simulink model "Simulacion_trayectoria"  (R2021a)
settings: Solver=VariableStepAuto  StartTime=0.0  StopTime=80  RelTol=1e-3
model workspace: external: MATLAB File G:\My Drive\0. PUCP\Cursos\2020.2\IEE243 - Sistemas de Control\Tarea Academica\Simulacion Robot Movil\cad files\RobotMovil_DataFile.m (data not in the file)
undefined symbols (not defined in the file): smiData, X, xPla, Y, yPla, Z, zPla
libraries: sm_lib x211, nesl_utility x6, simulink x3, fl_lib x3
(part 5 of 5)

== system Simulacion_trayectoria/MODELO CINEMÁTICO ROBOT MOVIL1/RobotMovilBase_2_RIGID/shield_rb_1_RIGID/shield_rb_step_1_RIGID/tc_3528_step_1_RIGID ==
  ReferenceFrame : sm_lib/Frames and Transforms/Reference Frame
  Solid : sm_lib/Body Elements/File Solid  ExtGeomFileName=tc_3528.step_Default_sldprt.STEP  UnitType=FromFile  ExtGeomFileUnits=m  StepReaderType=HEX  ExportConvexHullGeometry=off  InertiaType=Custom  Mass=smiData.Solid(7).mass  MassUnits=kg  CenterOfMass=smiData.Solid(7).CoM  CenterOfMassUnits=mm  MomentsOfInertia=smiData.Solid(7).MoI  MomentsOfInertiaUnits=kg*mm^2  ProductsOfInertia=smiData.Solid(7).PoI  ProductsOfInertiaUnits=kg*mm^2  BasedOnType=DensityFromFile  Density=1000  DensityUnits=kg/m^3  DoExposeReferenceFrame=on  SerializedFrames=<Frames/>  GraphicType=FromGeometry  MarkerShape=Sphere  MarkerSize=10  GraphicVisPropType=SimpleVisualProperties  GraphicDiffuseColor=smiData.Solid(7).color  GraphicSpecularColor=[0.5 0.5 0.5 1.0]  GraphicAmbientColor=[0.15 0.15 0.15 1.0]  GraphicEmissiveColor=[0.0 0.0 0.0 1.0]  GraphicShininess=75  GraphicOpacity=smiData.Solid(7).opacity
  F : PMIOPort  Side=Left
  connections:
  Solid/RConn1 -- ReferenceFrame/RConn1 -- F/RConn1

== matlab function Simulacion_trayectoria/Controlador de Seguimiento de Trayectoria1 ==
  data: xd input; yd input; xdp input; w_ref output; ydp input; x input; y input; u_ref output; phi input
function [w_ref, u_ref] = fcn(xd,yd,xdp,ydp,x,y,phi)

a = 0.147/2;
K1 = 16;%Tes=0.25 seg
K2 = 16;%Tes=0.25 seg
%phi en radianes
xa = x + a*cos(phi);
ya = y + a*sin(phi);
%definimos la matriz M
detM=a;
Minv_11 = a*cos(phi)/detM;
Minv_12 = a*sin(phi)/detM;
Minv_21 = -sin(phi)/detM;
Minv_22 = cos(phi)/detM;
%
av1 = xdp + K1*(xd-xa);
av2 = ydp + K2*(yd-ya);
%
u_ref = Minv_11*av1 + Minv_12*av2;
w_ref = Minv_21*av1 + Minv_22*av2;%está radianes

== matlab function Simulacion_trayectoria/MATLAB Function1 ==
  data: x input; xa output; y input; phi input; ya output
function [xa,ya] = fcn(x,y,phi)

a = 0.147/2;

xa = x + a*cos(phi);
ya = y + a*sin(phi);

== matlab function Simulacion_trayectoria/Trayectoria1 ==
  data: u input; xd output; yd output; xdp output; ydp output
function [xd,yd,xdp,ydp] = fcn(u)
%Son 14 caminos. Si el recorrido total dura 60 segundos, cada camino debe 
%demorar como mucho 4.2857 segundos(aproximamos a 4 segundos). Y dado que
%se desea que en "10 pasos" se pueda cumplir con un trayecto, el tiempo de 
%muestro de este bloque debe ser 0.4segundos.
persistent t
persistent xo
persistent yo
persistent camino_1
persistent camino_2
persistent camino_3
persistent camino_4
persistent camino_5
persistent camino_6
persistent camino_7
persistent camino_8
persistent camino_9
persistent camino_10
persistent camino_11
persistent camino_12
persistent camino_13

if isempty(t)
    t=0;
    xo=0.168;
    yo=0;
    camino_1=true;
    camino_2=true;
    camino_3=true;
    camino_4=true;
    camino_5=true;
    camino_6=true;
    camino_7=true;
    camino_8=true;
    camino_9=true;
    camino_10=true;
    camino_11=true;
    camino_12=true;
    camino_13=true;
end
if camino_1
    xd=xo+0.168*cosd(180-t);
    yd=yo+0.168*sind(180-t);
    %derivada
    xdp=0.168*sind(180-t);
    ydp=0.168*-cosd(180-t);
    if t>=128
        camino_1=false;
        %Añadimos el centro
        xo=xd+0.1*sind(38);
        yo=yd+0.1*cosd(38);
        t=0;
    else
        t = t + 12.8;     
    end
elseif camino_2
    xd=xo+0.1*cosd(-128+t);
    yd=yo+0.1*sind(-128+t);
    %derivada
    xdp=0.1*-sind(-128+t);
    ydp=0.1*cosd(-128+t);
    if t>=78
        camino_2=false;
        %Añadimos el centro
        xo=xd+0.168*sind(40);
        yo=yd-0.168*cosd(40);
        t=0;
    else
        t = t + 7.8;     
    end
elseif camino_3
    xd=xo+0.168*cosd(130-t);
    yd=yo+0.168*sind(130-t);
    %derivada
    xdp=0.168*sind(130-t);
    ydp=0.168*-cosd(130-t);
    if t>=68
        camino_3=false;
        %Añadimos el centro
        xo=xd+0.05*sind(28);
        yo=yd+0.05*cosd(28);
        t=0;
    else
        t = t + 6.8;     
    end   
elseif camino_4
    xd=xo+0.05*cosd(-118+t);
    yd=yo+0.05*sind(-118+t);
    %derivada
    xdp=0.05*-sind(-118+t);
    ydp=0.05*cosd(-118+t);
    if t>=137
        camino_4=false;
        %Añadimos el centro
        xo=xd-0.75*sind(71);
        yo=yd-0.75*cosd(71);
        t=0;
    else
        t = t + 13.7;     
    end
elseif camino_5
    xd=xo+0.75*cosd(19+t);
    yd=yo+0.75*sind(19+t);
    %derivada
    xdp=0.75*-sind(19+t);
    ydp=0.75*cosd(19+t);
    if t>=142
        camino_5=false;
        %Añadimos el centro
        xo=xd+0.05*cosd(19);
        yo=yd-0.05*cosd(19);
        t=0;
    else
        t = t + 14.2;     
    end   
elseif camino_6
    xd=xo+0.05*cosd(161+t);
    yd=yo+0.05*sind(161+t);
    %derivada
    xdp=0.05*-sind(161+t);
    ydp=0.05*cosd(161+t);
    if t>=137
        camino_6=false;
        %Añadimos el centro
        xo=xd+0.168*sind(28);
        yo=yd-0.168*cosd(28);
        t=0;
    else
        t = t + 13.7;     
    end
elseif camino_7
    xd=xo+0.168*cosd(118-t);
    yd=yo+0.168*sind(118-t);
    %derivada
    xdp=0.168*sind(118-t);
    ydp=0.168*-cosd(118-t);
    if t>=68    
        camino_7=false;
        %Añadimos el centro
        xo=xd+0.1*sind(40);
        yo=yd+0.1*cosd(40);
        t=0;
    else
        t = t + 6.8;     
    end   
elseif camino_8
    xd=xo+0.1*cosd(-130+t);
    yd=yo+0.1*sind(-130+t);
    %derivada
    xdp=0.1*-sind(-130+t);
    ydp=0.1*cosd(-130+t);
    if t>=78
        camino_8=false;
        %Añadimos el centro
        xo=xd+0.168*sind(38);
        yo=yd-0.168*cosd(38);
        t=0;
    else
        t = t + 7.8;     
    end
elseif camino_9
    xd=xo+0.168*cosd(128-t);
    yd=yo+0.168*sind(128-t);
    %derivada
    xdp=0.168*sind(180-t);
    ydp=0.168*-cosd(180-t);
    if t>=128
        camino_9=false;
        xo=xd;
        yo=yd;
        t=0;
    else
        t = t + 12.8;     
    end
elseif camino_10
    xd=xo;
    yd=yo+0.15*sind(-90)*t;
    xdp=0;
    ydp=0.15*sind(-90)*t;
    d_recorrida=0.15*t; %velocidad*tiempo
    t = t + 0.4;
    if d_recorrida>=0.6
        %añadir el centro
        camino_10=false;
        xo=xd+0.365;
        yo=yd;
        t=0;
    end
elseif camino_11 
    xd=xo+0.365*cosd(180+t);
    yd=yo+0.365*sind(180+t);
    %derivada
    xdp=0.365*-sind(180+t);
    ydp=0.365*cosd(180+t);
    if t>=166.56
        camino_11=false;
        %añadir el centro
        xo=xd-0.075*cosd(13.44);
        yo=yd+0.075*sind(13.44);
        t=0;
    else
        t = t + 16.656;     
    end
elseif camino_12
    xd=xo+0.075*cosd(-13.44+t);
    yd=yo+0.075*sind(-13.44+t);
    %derivada
    xdp=0.075*-sind(-13.44+t);
    ydp=0.075*cosd(-13.44+t);
    if t>=180
        camino_12=false;
        %añadir el centro
        xo=xd-0.215*cosd(13.44);
        yo=yd+0.215*sind(13.44);
        t=0;
    else
        t = t + 18;     
    end
elseif camino_13
    xd=xo+0.215*cosd(-13.44-t);
    yd=yo+0.215*sind(-13.44-t);
    %derivada
    xdp=0.215*sind(-13.44-t);
    ydp=0.215*-cosd(-13.44-t);
    if t>= 166.56
        camino_13=false;
        xo=xd;
        yo=yd;
        t=0;
    else
        t = t + 16.656;     
    end
else%if camino_14
    xd=xo;
    yd=yo+0.15*sind(90)*t;
    xdp=0;
    ydp=0.15*sind(90)*t;
    d_recorrida=0.15*t; %velocidad*tiempo
    t = t + 0.4;
    if d_recorrida>=0.6
        %camino_14=false;
        t=0;
        xo=0.168;
        yo=0;
        camino_1=true;
        camino_2=true;
        camino_3=true;
        camino_4=true;
        camino_5=true;
        camino_6=true;
        camino_7=true;
        camino_8=true;
        camino_9=true;
        camino_10=true;
        camino_11=true;
        camino_12=true;
        camino_13=true;
    end
end
%para reducir el tamaño de la estrella
% xd=xd/10;
% yd=yd/10;
% xdp=xdp/10;
% ydp=ydp/10;

== matlab function Simulacion_trayectoria/Control velocidad/Control Derecho/PI2 ==
  data: e input; u output
function u = fcn(e)

persistent ud_1
persistent ed_1
if isempty(ud_1)
    ud_1=0;
    ed_1=0;
end
Ts=0.01;
Kp = 0.0208;
Ki = 0.1248;
u=ud_1+(2*Kp+Ki*Ts)/2*e+(Ki*Ts-2*Kp)/2*ed_1;
ed_1=e;
ud_1=u;

== matlab function Simulacion_trayectoria/Control velocidad/Control izquierdo/PI2 ==
  data: e input; u output
function u = fcn(e)

persistent ui_1
persistent ei_1
if isempty(ui_1)
    ui_1=0;
    ei_1=0;
end
Ts=0.006;
Kp=0.020056241439231;
Ki=0.441237311663075;
u=ui_1+(2*Kp+Ki*Ts)/2*e+(Ki*Ts-2*Kp)/2*ei_1;
ei_1=e;
ui_1=u;
